simulink model "Kin_r_cc"  (R2015b)
settings: Solver=FixedStepDiscrete  StartTime=0.0  StopTime=28  FixedStep=0.010  RelTol=1e-3
PostLoadFcn:
  | , if any(exist('dsrtsu_mdlpostloadfcn', 'file') == [2, 3, 6]), try dsrtsu_mdlpostloadfcn('Execute', bdroot); catch fprintf('Error in PostLoadFcn (dsrtsu_mdlpostloadfcn) for model "%s":\n %s\n', bdroot, lasterr); end, end,
undefined symbols (not defined in the file or in its folder): BHA, CTRL, Data, DiscIntNeverNeededParam
libraries: libbha_kinematic_tools x6, libo_robotics x3, simulink x1
settings Model: DSRTSU_INTERNAL_RTI_VER=440  DSRTSU_INTERNAL_RTI_TYPE=rti1007  DSRTSU_INTERNAL_RTIFPGA=30  Creator=Mahl  LastModifiedBy=Mayer
settings DataIOCC: SaveFormat=Array
settings OptimizationCC: BlockReduction=off  OptimizeBlockIOStorage=off  BufferReuse=off  GlobalBufferReuse=off  ExpressionFolding=off  ExpressionDepthLimit=2147483647  LocalBlockOutputs=off
settings DebuggingCC: SolverPrmCheckMsg=warning  StateNameClashWarn=warning
settings HardwareCC: ProdBitPerPointer=32  ProdLargestAtomicFloat=None  ProdEndianess=BigEndian  ProdWordSize=32  ProdHWDeviceType=Generic->Custom  TargetIntDivRoundTo=Zero  TargetEndianess=BigEndian  TargetHWDeviceType=Generic->Custom
settings RTWCC: SystemTargetFile=rti1103.tlc  MakeCommand=make_rti  TemplateMakefile=rti1103.tmf  Description=dSPACE DS1103 Hardware Platform
settings STFCustomTargetCC: ParMdlRefBuildCompliant=on  ConcurrentExecutionCompliant=off  MatFileLogging=on  SystemTargetFile=rti1103.tlc
settings GRTTargetCC: CompOptLevelCompliant=off  ConcurrentExecutionCompliant=off  GeneratePreprocessorConditionals=Disable all  CombineOutputUpdateFcns=off  GRTInterface=on  UseToolchainInfoCompliant=off  ExtModeMexFile=noextcomm
settings ConfigComp: CovModelRefEnable=Off

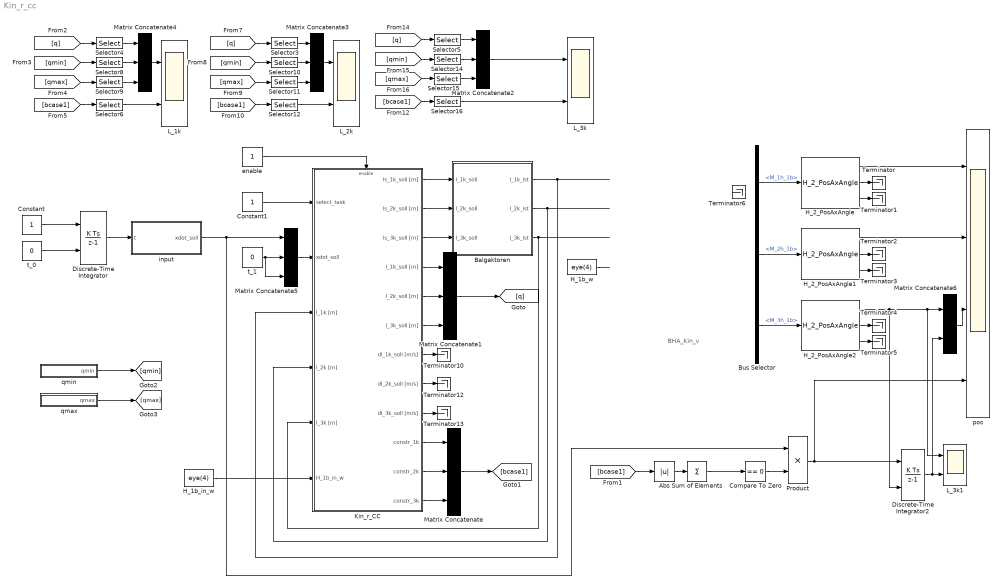
== system Kin_r_cc ==
  note: BHA_Kin_v
  Abs : Abs
  Balgaktoren : Subsystem
  Bus Selector : BusSelector  OutputSignals=Section1.M_1h_1b,Section2.M_2h_1b,Section3.M_3h_1b
  Compare To Zero : simulink/Logic and Bit Operations/Compare To Zero  relop===  OutDataTypeStr=uint8
  Constant : Constant
  Constant1 : Constant
  Discrete-Time Integrator : DiscreteIntegrator  InitialConditionSource=external  InitialConditionSetting=State (most efficient)  SampleTime=0.010  ICPrevOutput=DiscIntNeverNeededParam  ICPrevScaledInput=DiscIntNeverNeededParam
  Discrete-Time Integrator2 : DiscreteIntegrator  InitialConditionSource=external  InitialConditionSetting=State (most efficient)  SampleTime=-1  ICPrevOutput=DiscIntNeverNeededParam  ICPrevScaledInput=DiscIntNeverNeededParam
  H_1b_in_w : Constant  Value=eye(4)
  H_1b_w : Constant  Value=eye(4)
  H_2_PosAxAngle : libo_robotics/Kinematics/H_2_PosAxAngle
  H_2_PosAxAngle1 : libo_robotics/Kinematics/H_2_PosAxAngle
  H_2_PosAxAngle2 : libo_robotics/Kinematics/H_2_PosAxAngle
  Kin_r_CC : Subsystem
  L_1k : Scope  NumInputPorts=2
  L_2k : Scope  NumInputPorts=2
  L_3k : Scope  NumInputPorts=2
  L_3k1 : Scope  NumInputPorts=2
  Matrix Concatenate{,1..5} (6 alike) : Concatenate  NumInputs=3  Mode=Multidimensional array
  Matrix Concatenate6 : Concatenate  Mode=Multidimensional array
  Product : Product  RndMeth=Zero
  Selector{3,10..12} (4 alike) : Selector  InputPortWidth=9  IndexOptions=Index vector (dialog)  Indices=[4:6]  OutputSizes=1
      settings: AttributesFormatString=out: %<Indices>
  Selector{5,14..16} (4 alike) : Selector  InputPortWidth=9  IndexOptions=Index vector (dialog)  Indices=[7:9]  OutputSizes=1
      settings: AttributesFormatString=out: %<Indices>
  Selector{4,6,8..9} (4 alike) : Selector  InputPortWidth=9  IndexOptions=Index vector (dialog)  Indices=[1:3]  OutputSizes=1
      settings: AttributesFormatString=out: %<Indices>
  Sum of Elements : Sum  Inputs=+
  Terminator{,1..6,10,12..13} (10 alike) : Terminator
  enable : Constant
  input : Subsystem
  pos : Scope  NumInputPorts=4
  qmax : Subsystem
  qmin : Subsystem
  t_0 : Constant  Value=0
  t_1 : Constant  Value=0
  wires:
  Discrete-Time Integrator/1 -> input/1(t)
  Constant/1 -> Discrete-Time Integrator/1
  t_0/1 -> Discrete-Time Integrator/2
  H_1b_w/1 -> ?
  ? -> Bus Selector/1
  Bus Selector/1 -> H_2_PosAxAngle/1  "<M_1h_1b>"
  Bus Selector/2 -> H_2_PosAxAngle1/1  "<M_2h_1b>"
  Bus Selector/3 -> H_2_PosAxAngle2/1  "<M_3h_1b>"
  H_2_PosAxAngle/1 -> pos/1
  H_2_PosAxAngle1/1 -> pos/2
  H_2_PosAxAngle2/1 -> Matrix Concatenate6/1, L_3k1/1, Discrete-Time Integrator2/2
  Selector4/1 -> Matrix Concatenate4/1
  Selector6/1 -> L_1k/2
  Selector8/1 -> Matrix Concatenate4/2
  Selector9/1 -> Matrix Concatenate4/3
  Selector3/1 -> Matrix Concatenate3/1
  Selector12/1 -> L_2k/2
  Selector10/1 -> Matrix Concatenate3/2
  Selector11/1 -> Matrix Concatenate3/3
  Selector5/1 -> Matrix Concatenate2/1
  Selector16/1 -> L_3k/2
  Selector14/1 -> Matrix Concatenate2/2
  Selector15/1 -> Matrix Concatenate2/3
  H_2_PosAxAngle/2 -> Terminator/1
  H_2_PosAxAngle/3 -> Terminator1/1
  H_2_PosAxAngle1/2 -> Terminator2/1
  H_2_PosAxAngle1/3 -> Terminator3/1
  H_2_PosAxAngle2/2 -> Terminator4/1
  H_2_PosAxAngle2/3 -> Terminator5/1
  ? -> Terminator6/1
  Kin_r_CC/1(ls_1k_soll [m]) -> Balgaktoren/1(l_1k_soll)
  Kin_r_CC/2(ls_2k_soll [m]) -> Balgaktoren/2(l_2k_soll)
  Kin_r_CC/3(ls_3k_soll [m]) -> Balgaktoren/3(l_3k_soll)
  Balgaktoren/1(l_1k_ist) -> Kin_r_CC/3(l_1k [m])
  Balgaktoren/2(l_2k_ist) -> Kin_r_CC/4(l_2k [m])
  Balgaktoren/3(l_3k_ist) -> Kin_r_CC/5(l_3k [m])
  Compare To Zero/1 -> Product/2
  Product/1 -> Discrete-Time Integrator2/1, pos/4
  Discrete-Time Integrator2/1 -> Matrix Concatenate6/2, L_3k1/2
  [q] -> Selector4/1
  [qmin] -> Selector8/1
  [qmax] -> Selector9/1
  [bcase1] -> Selector6/1
  [q] -> Selector3/1
  [qmin] -> Selector10/1
  [qmax] -> Selector11/1
  [bcase1] -> Selector12/1
  [q] -> Selector5/1
  [qmin] -> Selector14/1
  [qmax] -> Selector15/1
  [bcase1] -> Selector16/1
  input/1(xdot_soll) -> Matrix Concatenate5/1, Product/1
  Kin_r_CC/4(l_1k_soll [m]) -> Matrix Concatenate1/1
  Kin_r_CC/5(l_2k_soll [m]) -> Matrix Concatenate1/2
  Kin_r_CC/6(l_3k_soll [m]) -> Matrix Concatenate1/3
  Kin_r_CC/7(dl_1k_soll [m/s]) -> Terminator10/1
  Kin_r_CC/8(dl_2k_soll [m/s]) -> Terminator12/1
  Kin_r_CC/9(dl_3k_soll [m/s]) -> Terminator13/1
  Kin_r_CC/10(constr_1k) -> Matrix Concatenate/1
  Kin_r_CC/11(constr_2k) -> Matrix Concatenate/2
  Kin_r_CC/12(constr_3k) -> Matrix Concatenate/3
  H_1b_in_w/1 -> Kin_r_CC/6(H_1b_in_w)
  qmin/1(qmin) -> [qmin]
  qmax/1(qmax) -> [qmax]
  Constant1/1 -> Kin_r_CC/1(select_task)
  Matrix Concatenate5/1 -> Kin_r_CC/2(xdot_soll)
  t_1/1 -> Matrix Concatenate5/2, Matrix Concatenate5/3
  enable/1 -> Kin_r_CC/Enable
  Matrix Concatenate/1 -> [bcase1]
  [bcase1] -> Abs/1
  Abs/1 -> Sum of Elements/1
  Sum of Elements/1 -> Compare To Zero/1
  Matrix Concatenate1/1 -> [q]
  Matrix Concatenate2/1 -> L_3k/1
  Matrix Concatenate3/1 -> L_2k/1
  Matrix Concatenate4/1 -> L_1k/1
  Matrix Concatenate6/1 -> pos/3

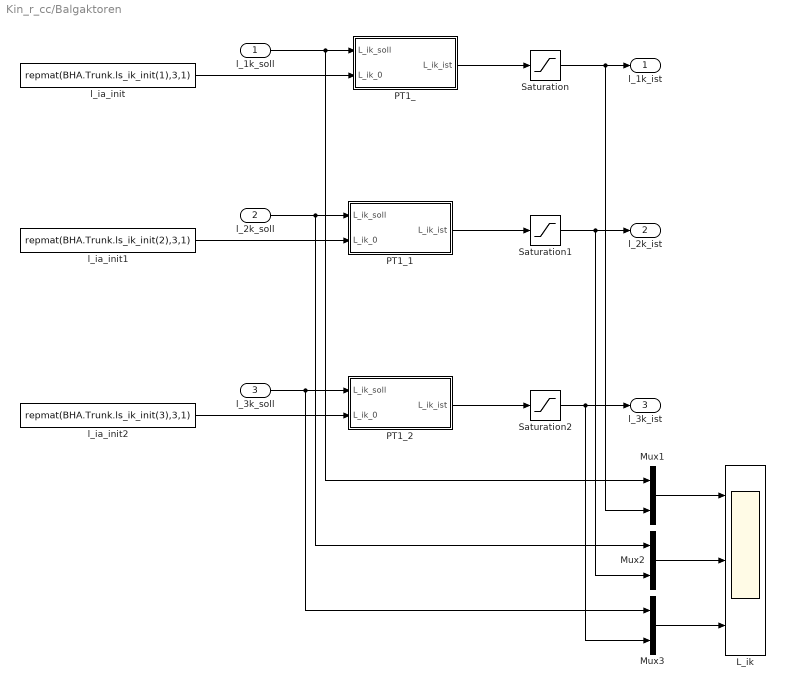
== system Kin_r_cc/Balgaktoren ==
  l_1k_soll : Inport
  l_2k_soll : Inport  Port=2
  l_3k_soll : Inport  Port=3
  L_ik : Scope  NumInputPorts=3
  Mux1 : Mux  Inputs=2
  Mux2 : Mux  Inputs=2
  Mux3 : Mux  Inputs=2
  PT1_ : Subsystem
  PT1_1 : Subsystem
  PT1_2 : Subsystem
  Saturation : Saturate  UpperLimit=inf  LowerLimit=BHA.Trunk.ls_ik_min(1)
  Saturation1 : Saturate  UpperLimit=inf  LowerLimit=BHA.Trunk.ls_ik_min(2)
  Saturation2 : Saturate  UpperLimit=inf  LowerLimit=BHA.Trunk.ls_ik_min(3)
  l_ia_init : Constant  Value=repmat(BHA.Trunk.ls_ik_init(1),3,1)
  l_ia_init1 : Constant  Value=repmat(BHA.Trunk.ls_ik_init(2),3,1)
  l_ia_init2 : Constant  Value=repmat(BHA.Trunk.ls_ik_init(3),3,1)
  l_1k_ist : Outport
  l_2k_ist : Outport  Port=2
  l_3k_ist : Outport  Port=3
  wires:
  l_1k_soll/1 -> PT1_/1(L_ik_soll), Mux1/1
  l_2k_soll/1 -> PT1_1/1(L_ik_soll), Mux2/1
  l_3k_soll/1 -> PT1_2/1(L_ik_soll), Mux3/1
  PT1_/1(L_ik_ist) -> Saturation/1
  PT1_1/1(L_ik_ist) -> Saturation1/1
  PT1_2/1(L_ik_ist) -> Saturation2/1
  l_ia_init/1 -> PT1_/2(L_ik_0)
  l_ia_init1/1 -> PT1_1/2(L_ik_0)
  Saturation/1 -> l_1k_ist/1, Mux1/2
  Saturation1/1 -> l_2k_ist/1, Mux2/2
  Saturation2/1 -> l_3k_ist/1, Mux3/2
  l_ia_init2/1 -> PT1_2/2(L_ik_0)
  Mux1/1 -> L_ik/1
  Mux2/1 -> L_ik/2
  Mux3/1 -> L_ik/3

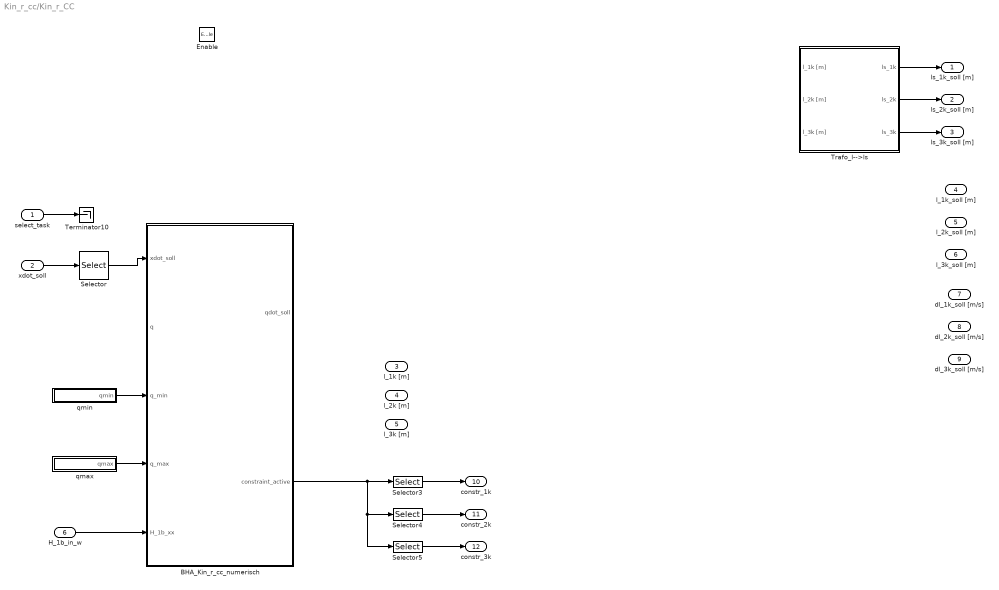
== system Kin_r_cc/Kin_r_CC ==
  select_task : Inport
  xdot_soll : Inport  Port=2
  l_1k [m] : Inport  Port=3
  l_2k [m] : Inport  Port=4
  l_3k [m] : Inport  Port=5
  H_1b_in_w : Inport  Port=6
  Enable : EnablePort  StatesWhenEnabling=reset
  BHA_Kin_r_cc_numerisch : Subsystem
  Selector : Selector  InputPortWidth=5  IndexOptions=Index vector (dialog)  Indices=[1 2 3]  OutputSizes=1
  Selector3 : Selector  InputPortWidth=9  IndexOptions=Index vector (dialog)  Indices=[1:3]  OutputSizes=1
      settings: AttributesFormatString=out: %<Indices>
  Selector4 : Selector  InputPortWidth=9  IndexOptions=Index vector (dialog)  Indices=[4:6]  OutputSizes=1
      settings: AttributesFormatString=out: %<Indices>
  Selector5 : Selector  InputPortWidth=9  IndexOptions=Index vector (dialog)  Indices=[7:9]  OutputSizes=1
      settings: AttributesFormatString=out: %<Indices>
  Terminator10 : Terminator
  Trafo_l-->ls : Subsystem
  qmax : Subsystem
  qmin : Subsystem
  ls_1k_soll [m] : Outport
  ls_2k_soll [m] : Outport  Port=2
  ls_3k_soll [m] : Outport  Port=3
  l_1k_soll [m] : Outport  Port=4
  l_2k_soll [m] : Outport  Port=5
  l_3k_soll [m] : Outport  Port=6
  dl_1k_soll [m/s] : Outport  Port=7
  dl_2k_soll [m/s] : Outport  Port=8
  dl_3k_soll [m/s] : Outport  Port=9
  constr_1k : Outport  Port=10
  constr_2k : Outport  Port=11
  constr_3k : Outport  Port=12
  wires:
  Selector5/1 -> constr_3k/1
  Selector4/1 -> constr_2k/1
  Selector3/1 -> constr_1k/1
  BHA_Kin_r_cc_numerisch/2(constraint_active) -> Selector3/1, Selector4/1, Selector5/1
  ? -> dl_3k_soll [m/s]/1
  ? -> dl_2k_soll [m/s]/1
  ? -> dl_1k_soll [m/s]/1
  ? -> l_3k_soll [m]/1
  ? -> l_2k_soll [m]/1
  ? -> l_1k_soll [m]/1
  H_1b_in_w/1 -> BHA_Kin_r_cc_numerisch/5(H_1b_xx)
  select_task/1 -> Terminator10/1
  xdot_soll/1 -> Selector/1
  qmin/1(qmin) -> BHA_Kin_r_cc_numerisch/3(q_min)
  qmax/1(qmax) -> BHA_Kin_r_cc_numerisch/4(q_max)
  Selector/1 -> BHA_Kin_r_cc_numerisch/1(xdot_soll)
  Trafo_l-->ls/3(ls_3k) -> ls_3k_soll [m]/1
  Trafo_l-->ls/2(ls_2k) -> ls_2k_soll [m]/1
  Trafo_l-->ls/1(ls_1k) -> ls_1k_soll [m]/1

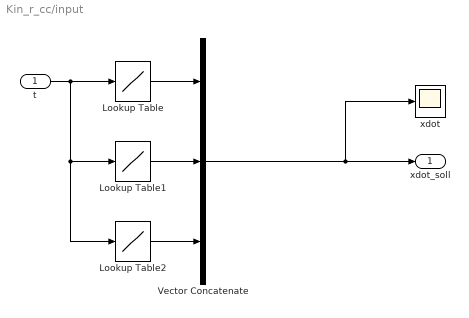
== system Kin_r_cc/input ==
  t : Inport
  Lookup Table : Lookup_n-D  NumberOfTableDimensions=1  BreakpointsForDimension1=Data.time  Table=Data.xdot_soll(1,:)  InterpMethod=Flat  ExtrapMethod=Clip  InternalRulePriority=Speed  InputSameDT=on
      settings: AttributesFormatString=%<Table>
  Lookup Table1 : Lookup_n-D  NumberOfTableDimensions=1  BreakpointsForDimension1=Data.time  Table=Data.ydot_soll(1,:)  InterpMethod=Flat  ExtrapMethod=Clip  InternalRulePriority=Speed  InputSameDT=on
      settings: AttributesFormatString=%<Table>
  Lookup Table2 : Lookup_n-D  NumberOfTableDimensions=1  BreakpointsForDimension1=Data.time  Table=Data.zdot_soll(1,:)  InterpMethod=Flat  ExtrapMethod=Clip  InternalRulePriority=Speed  InputSameDT=on
      settings: AttributesFormatString=%<Table>
  Vector Concatenate : Concatenate  NumInputs=3  Mode=Multidimensional array
  xdot : Scope
  xdot_soll : Outport
  wires:
  t/1 -> Lookup Table2/1, Lookup Table1/1, Lookup Table/1
  Lookup Table/1 -> Vector Concatenate/1
  Lookup Table1/1 -> Vector Concatenate/2
  Lookup Table2/1 -> Vector Concatenate/3
  Vector Concatenate/1 -> xdot_soll/1, xdot/1

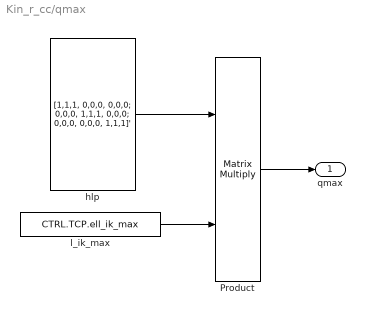
== system Kin_r_cc/qmax ==
  Product : Product  Multiplication=Matrix(*)  RndMeth=Zero
  hlp : Constant  Value=[1,1,1, 0,0,0, 0,0,0; 0,0,0, 1,1,1, 0,0,0; 0,0,0, 0,0,0, 1,1,1]'
  l_ik_max : Constant  Value=CTRL.TCP.ell_ik_max  VectorParams1D=off
  qmax : Outport
  wires:
  l_ik_max/1 -> Product/2
  hlp/1 -> Product/1
  Product/1 -> qmax/1

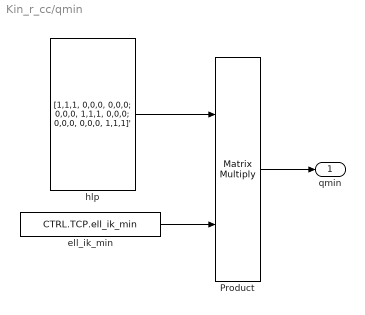
== system Kin_r_cc/qmin ==
  Product : Product  Multiplication=Matrix(*)  RndMeth=Zero
  ell_ik_min : Constant  Value=CTRL.TCP.ell_ik_min  VectorParams1D=off
  hlp : Constant  Value=[1,1,1, 0,0,0, 0,0,0; 0,0,0, 1,1,1, 0,0,0; 0,0,0, 0,0,0, 1,1,1]'
  qmin : Outport
  wires:
  Product/1 -> qmin/1
  hlp/1 -> Product/1
  ell_ik_min/1 -> Product/2

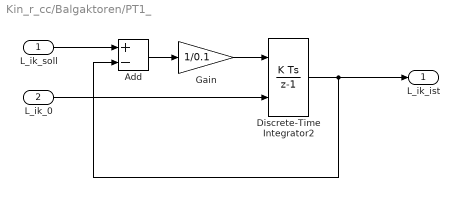
== system Kin_r_cc/Balgaktoren/PT1_ ==
  L_ik_soll : Inport
  L_ik_0 : Inport  Port=2
  Add : Sum  Inputs=+-
  Discrete-Time Integrator2 : DiscreteIntegrator  InitialConditionSource=external  InitialConditionSetting=State (most efficient)  SampleTime=-1  ICPrevOutput=DiscIntNeverNeededParam  ICPrevScaledInput=DiscIntNeverNeededParam
  Gain : Gain  Gain=1/0.1
  L_ik_ist : Outport
  wires:
  L_ik_soll/1 -> Add/1
  Discrete-Time Integrator2/1 -> Add/2, L_ik_ist/1
  Add/1 -> Gain/1
  Gain/1 -> Discrete-Time Integrator2/1
  L_ik_0/1 -> Discrete-Time Integrator2/2

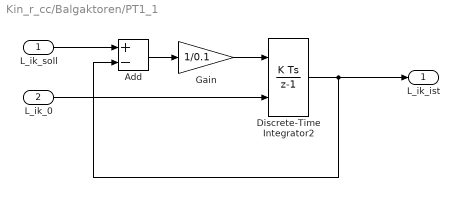
== system Kin_r_cc/Balgaktoren/PT1_1 ==
  L_ik_soll : Inport
  L_ik_0 : Inport  Port=2
  Add : Sum  Inputs=+-
  Discrete-Time Integrator2 : DiscreteIntegrator  InitialConditionSource=external  InitialConditionSetting=State (most efficient)  SampleTime=-1  ICPrevOutput=DiscIntNeverNeededParam  ICPrevScaledInput=DiscIntNeverNeededParam
  Gain : Gain  Gain=1/0.1
  L_ik_ist : Outport
  wires:
  L_ik_0/1 -> Discrete-Time Integrator2/2
  Gain/1 -> Discrete-Time Integrator2/1
  Add/1 -> Gain/1
  Discrete-Time Integrator2/1 -> L_ik_ist/1, Add/2
  L_ik_soll/1 -> Add/1

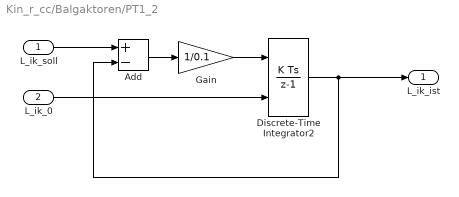
== system Kin_r_cc/Balgaktoren/PT1_2 ==
  L_ik_soll : Inport
  L_ik_0 : Inport  Port=2
  Add : Sum  Inputs=+-
  Discrete-Time Integrator2 : DiscreteIntegrator  InitialConditionSource=external  InitialConditionSetting=State (most efficient)  SampleTime=-1  ICPrevOutput=DiscIntNeverNeededParam  ICPrevScaledInput=DiscIntNeverNeededParam
  Gain : Gain  Gain=1/0.1
  L_ik_ist : Outport
  wires:
  L_ik_soll/1 -> Add/1
  Discrete-Time Integrator2/1 -> Add/2, L_ik_ist/1
  Add/1 -> Gain/1
  Gain/1 -> Discrete-Time Integrator2/1
  L_ik_0/1 -> Discrete-Time Integrator2/2

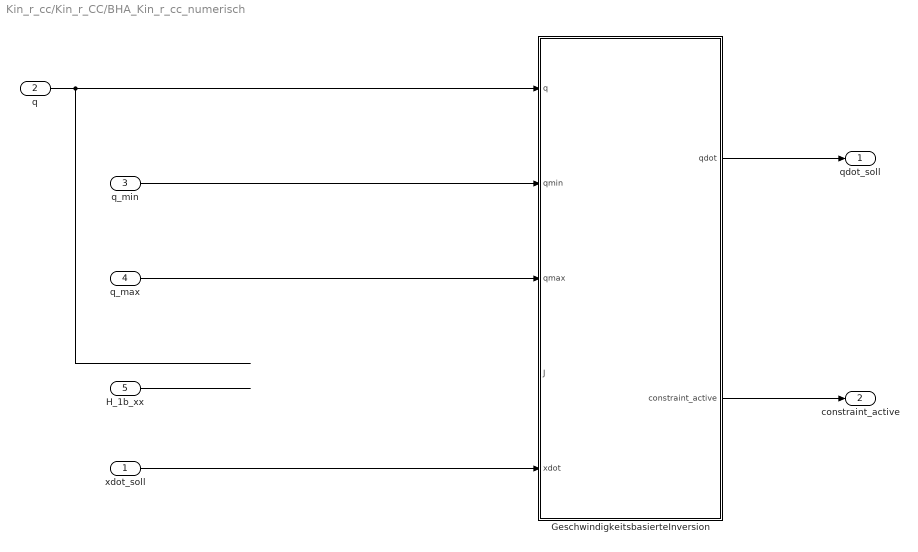
== system Kin_r_cc/Kin_r_CC/BHA_Kin_r_cc_numerisch ==
  xdot_soll : Inport
  q : Inport  Port=2
  q_min : Inport  Port=3
  q_max : Inport  Port=4
  H_1b_xx : Inport  Port=5
  GeschwindigkeitsbasierteInversion : Subsystem
  qdot_soll : Outport
  constraint_active : Outport  Port=2
  wires:
  H_1b_xx/1 -> ?
  q_max/1 -> GeschwindigkeitsbasierteInversion/3(qmax)
  q_min/1 -> GeschwindigkeitsbasierteInversion/2(qmin)
  q/1 -> GeschwindigkeitsbasierteInversion/1(q)
  xdot_soll/1 -> GeschwindigkeitsbasierteInversion/5(xdot)
  GeschwindigkeitsbasierteInversion/2(constraint_active) -> constraint_active/1
  GeschwindigkeitsbasierteInversion/1(qdot) -> qdot_soll/1
  ? -> GeschwindigkeitsbasierteInversion/4(J)

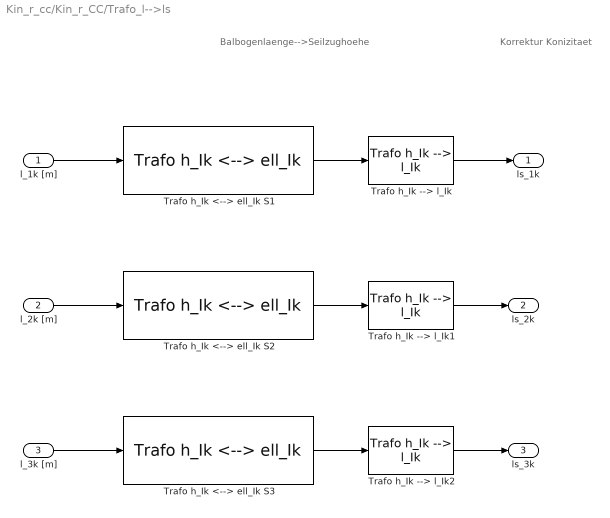
== system Kin_r_cc/Kin_r_CC/Trafo_l-->ls ==
  note: Korrektur Konizitaet
  note: Balbogenlaenge-->Seilzughoehe
  l_1k [m] : Inport
  l_2k [m] : Inport  Port=2
  l_3k [m] : Inport  Port=3
  Trafo h_Ik --> l_Ik : libbha_kinematic_tools/Trafo h_Ik --> l_Ik  ii=1 = gross
      settings: AttributesFormatString=Seilzughöhe > Seilzuglänge\nSektion = %<ii>
  Trafo h_Ik --> l_Ik1 : libbha_kinematic_tools/Trafo h_Ik --> l_Ik  ii=2 = mittel
      settings: AttributesFormatString=Seilzughöhe > Seilzuglänge\nSektion = %<ii>
  Trafo h_Ik --> l_Ik2 : libbha_kinematic_tools/Trafo h_Ik --> l_Ik  ii=3 = klein
      settings: AttributesFormatString=Seilzughöhe > Seilzuglänge\nSektion = %<ii>
  Trafo h_Ik <--> ell_Ik S1 : libbha_kinematic_tools/Trafo h_Ik <--> ell_Ik  inv=off  ii=1  m_i=BHA.Trunk.vc.num_segm  r_Si=BHA.Trunk.r_ms_i  r_Ai=BHA.Trunk.r_mb_i
      settings: AttributesFormatString=Seilzughöhe <> Balgbogenlänge\ninv = %<inv> | Sektion %<ii>
  Trafo h_Ik <--> ell_Ik S2 : libbha_kinematic_tools/Trafo h_Ik <--> ell_Ik  inv=off  ii=1  m_i=BHA.Trunk.vc.num_segm  r_Si=BHA.Trunk.r_ms_i  r_Ai=BHA.Trunk.r_mb_i
      settings: AttributesFormatString=Seilzughöhe <> Balgbogenlänge\ninv = %<inv> | Sektion %<ii>
  Trafo h_Ik <--> ell_Ik S3 : libbha_kinematic_tools/Trafo h_Ik <--> ell_Ik  inv=off  ii=3  m_i=BHA.Trunk.vc.num_segm  r_Si=BHA.Trunk.r_ms_i  r_Ai=BHA.Trunk.r_mb_i
      settings: AttributesFormatString=Seilzughöhe <> Balgbogenlänge\ninv = %<inv> | Sektion %<ii>
  ls_1k : Outport
  ls_2k : Outport  Port=2
  ls_3k : Outport  Port=3
  wires:
  Trafo h_Ik --> l_Ik2/1 -> ls_3k/1
  Trafo h_Ik --> l_Ik1/1 -> ls_2k/1
  Trafo h_Ik --> l_Ik/1 -> ls_1k/1
  Trafo h_Ik <--> ell_Ik S1/1 -> Trafo h_Ik --> l_Ik/1
  l_1k [m]/1 -> Trafo h_Ik <--> ell_Ik S1/1
  l_2k [m]/1 -> Trafo h_Ik <--> ell_Ik S2/1
  l_3k [m]/1 -> Trafo h_Ik <--> ell_Ik S3/1
  Trafo h_Ik <--> ell_Ik S2/1 -> Trafo h_Ik --> l_Ik1/1
  Trafo h_Ik <--> ell_Ik S3/1 -> Trafo h_Ik --> l_Ik2/1

== system Kin_r_cc/Kin_r_CC/qmax ==
  Product : Product  Multiplication=Matrix(*)  RndMeth=Zero
  hlp : Constant  Value=[1,1,1, 0,0,0, 0,0,0; 0,0,0, 1,1,1, 0,0,0; 0,0,0, 0,0,0, 1,1,1]'
  l_ik_max : Constant  Value=CTRL.TCP.ell_ik_max  VectorParams1D=off
  qmax : Outport
  wires:
  Product/1 -> qmax/1
  hlp/1 -> Product/1
  l_ik_max/1 -> Product/2

== system Kin_r_cc/Kin_r_CC/qmin ==
  Product : Product  Multiplication=Matrix(*)  RndMeth=Zero
  ell_ik_min : Constant  Value=CTRL.TCP.ell_ik_min  VectorParams1D=off
  hlp : Constant  Value=[1,1,1, 0,0,0, 0,0,0; 0,0,0, 1,1,1, 0,0,0; 0,0,0, 0,0,0, 1,1,1]'
  qmin : Outport
  wires:
  ell_ik_min/1 -> Product/2
  hlp/1 -> Product/1
  Product/1 -> qmin/1

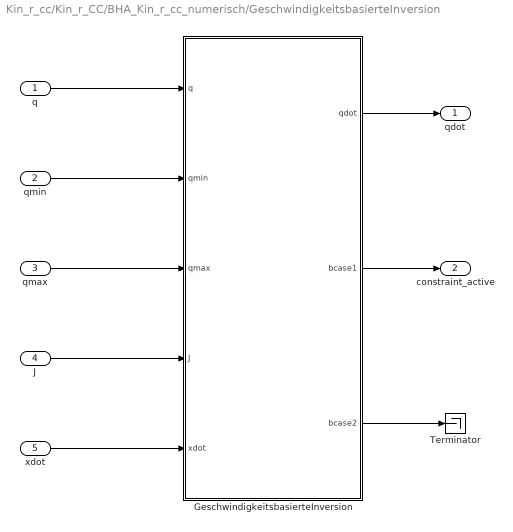
== system Kin_r_cc/Kin_r_CC/BHA_Kin_r_cc_numerisch/GeschwindigkeitsbasierteInversion ==
  q : Inport
  qmin : Inport  Port=2
  qmax : Inport  Port=3
  J : Inport  Port=4
  xdot : Inport  Port=5
  GeschwindigkeitsbasierteInversion : MATLAB Function  TreatAsAtomicUnit=on
  Terminator : Terminator
  qdot : Outport
  constraint_active : Outport  Port=2
  wires:
  GeschwindigkeitsbasierteInversion/3(bcase2) -> Terminator/1
  GeschwindigkeitsbasierteInversion/1(qdot) -> qdot/1
  GeschwindigkeitsbasierteInversion/2(bcase1) -> constraint_active/1
  xdot/1 -> GeschwindigkeitsbasierteInversion/5(xdot)
  J/1 -> GeschwindigkeitsbasierteInversion/4(J)
  qmax/1 -> GeschwindigkeitsbasierteInversion/3(qmax)
  qmin/1 -> GeschwindigkeitsbasierteInversion/2(qmin)
  q/1 -> GeschwindigkeitsbasierteInversion/1(q)

== matlab function Kin_r_cc/Kin_r_CC/BHA_Kin_r_cc_numerisch/GeschwindigkeitsbasierteInversion/GeschwindigkeitsbasierteInversion ==
  data: q input; qdot output; qmin input; qmax input; J input; xdot input; bcase1 output; bcase2 output
function [qdot, bcase1, bcase2]  = Kin_r(q, qmin, qmax, J, xdot)

% Input:
% q     [3n x 1]  Zustandsvektor Gelenkkoordinaten
% qmin  [3n x 1]  Minimalwert der Gelenkkoordinaten
% qmax  [3n x 1]  Maximalwert der Gelenkkoordinaten
% J(q)  [p x 3n]  Jacobi-Matrix
% xdot  [3 x 1]   Ableitung der Soll-Aufgabenkoordinaten
% eta   [1 x 1]   Halbe Ordnung des Strafpolynoms
%
% Output:
% qdot  [3n x 1]   Sollgeschwindigkeit der Gelenkkoordinaten
% bcase [3n x 1]   Zustand aktiver Stellgroessenbeschraenkungen
n=3;
p=3;
eta=4;

qdot    = zeros(3*n,1);    

%% Anteil der Gelenkgeschwindigkeit berechnet mit Moore-Penrose-Pseudoinverse
Jt      = J'*((J*J')\eye(p));
qdot1   = Jt*xdot;

%% Anteil der Gelenkgeschwindigkeit berechnet mit Gradient Projection Method
if(eta==0)
    qdot2   = zeros(3*n,1);
else
    q_m     = (qmin+qmax)/2;
    q_delta = (qmax-qmin)/2;
    q0dot   = -2*eta*((q-q_m)./q_delta).^(2*eta-1)./(3*n*q_delta);
    
    q0dot_b   = zeros(3*n,1);
    if norm(q0dot)>1e-9
        q0dot_b   = min(5*norm(qdot1)/norm(q0dot), 1)*q0dot;
    end
   
    qdot2   = (eye(3*n)-Jt*J)*q0dot_b;
end

%% Einhaltung von Beschraenkungen des Gelenkzustands
bcase1 = zeros(3*n,1);
bcase2 = zeros(3*n,1);
for ii = 1:3*n
    ccase = (qmax(ii)-q(ii)<=0) - (q(ii)-qmin(ii)<=0);
    if ccase<0
        if qdot1(ii)<0
            bcase1(ii) = -1;
        end
        if qdot2(ii)<0
            bcase2(ii) = -1;
        end
    end
    if ccase>0
        if qdot1(ii)>0
            bcase1(ii) = 1;
        end
        if qdot2(ii)>0
            bcase2(ii) = 1;
        end
    end        
end

if sum(abs(bcase1)) > 0
    qdot1 = zeros(3*n,1);
end
if sum(abs(bcase2)) > 0
    qdot2 = zeros(3*n,1);
end

%% Zusammenfassung beider Anteile
qdot = qdot1+qdot2;
